simulink model "Resp"  (R2024b)
settings: Solver=ode15s  StartTime=0  StopTime=30  MaxStep=1e-3  RelTol=1e-3
libraries: slpidlib x1
settings Model: Creator=piqui
settings DataIOCC: ReturnWorkspaceOutputs=off  TimeSaveName=t
settings DebuggingCC: AlgebraicLoopMsg=none  ArtificialAlgebraicLoopMsg=none  MaxConsecutiveZCsMsg=none  OperatingPointInterfaceChecksumMismatchMsg=none
settings RTWCC: GPUComputeCapability=3.5

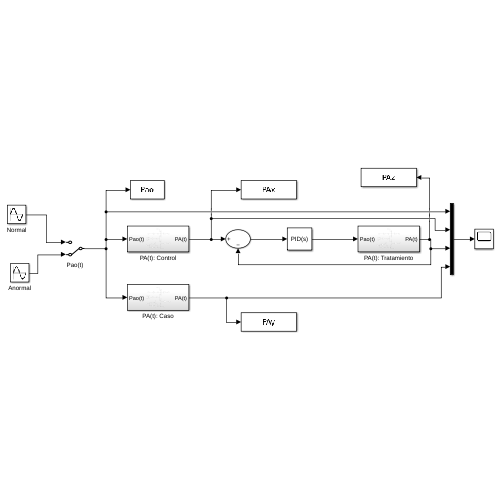
[thumbnail: Simulink's stored preview of the top-level diagram]
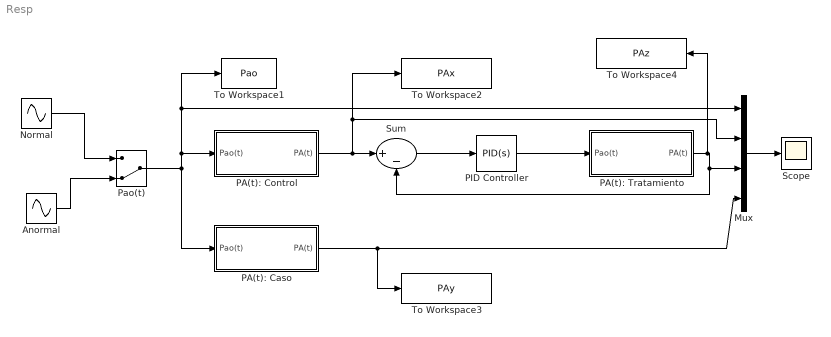
== system Resp ==
  Anormal : Sin  Amplitude=1.5  Frequency=pi/2  SampleTime=0
  Mux : Mux
  Normal : Sin  Amplitude=2.5  Frequency=pi  SampleTime=0
  PA(t): Caso : Subsystem
  PA(t): Control : Subsystem
  PA(t): Tratamiento : Subsystem
  PID Controller : slpidlib/PID Controller  Controller=PID  Form=Parallel  TimeDomain=Continuous-time  UseExternalTs=off  SampleTime=-1  IntegratorMethod=Forward Euler  FilterMethod=Forward Euler  ControllerParametersSource=internal  P=1511.4945  I=74979.6737  UseKiTs=off  D=7.0888  UseExternalDerivativeSource=off  N=55877.0023696936  UseFilter=on  TunerSelectOption=Transfer Function Based (PID Tuner App)  InitialConditionSource=internal  InitialConditionForIntegrator=0  InitialConditionForFilter=0  DifferentiatorICPrevScaledInput=0  ExternalReset=none  TrackingMode=off  Kt=1  LimitOutput=off  SatLimitsSource=internal  UpperSaturationLimit=inf  LowerSaturationLimit=-inf  LinearizeAsGain=on  AntiWindupMode=none  Kb=1  LimitIntegrator=off  UpperIntegratorSaturationLimit=inf  LowerIntegratorSaturationLimit=-inf  POutMin=[]  POutMax=[]  IOutMin=[]  IOutMax=[]  DOutMin=[]  DOutMax=[]  NOutMin=[]  NOutMax=[]  SumOutMin=[]  SumOutMax=[]  SaturationOutMin=[]  SaturationOutMax=[]  PParamMin=[]  PParamMax=[]  IParamMin=[]  IParamMax=[]  DParamMin=[]  DParamMax=[]  NParamMin=[]  NParamMax=[]  KbParamMin=[]  KbParamMax=[]  KtParamMin=[]  KtParamMax=[]  KbOutMin=[]  KbOutMax=[]  KtOutMin=[]  KtOutMax=[]  IntegratorOutMin=[]  IntegratorOutMax=[]  FilterOutMin=[]  FilterOutMax=[]  SumI1OutMin=[]  SumI1OutMax=[]  SumI2OutMin=[]  SumI2OutMax=[]  SumI3OutMin=[]  SumI3OutMax=[]  SumI4OutMin=[]  SumI4OutMax=[]  SumDOutMin=[]  SumDOutMax=[]  DifferentiatorOutMin=[]  DifferentiatorOutMax=[]  FilterDiffOutCoefMin=[]  FilterDiffOutCoefMax=[]  ReciprocalOutMin=[]  ReciprocalOutMax=[]  SumDenOutMin=[]  SumDenOutMax=[]  SumNumOutMin=[]  SumNumOutMax=[]  DivideOutMin=[]  DivideOutMax=[]  UdiffTsProdOutMin=[]  UdiffTsProdOutMax=[]  NTsProdOutMin=[]  NTsProdOutMax=[]  UintegralTsProdOutMin=[]  UintegralTsProdOutMax=[]  UngainTsProdOutMin=[]  UngainTsProdOutMax=[]  ClampingZeroOutDataTypeStr=Inherit: Inherit via back propagation  ClampingZeroOutMin=[]  ClampingZeroOutMax=[]  FilterDenConstantOutDataTypeStr=Inherit: Inherit via back propagation  FilterDenConstantOutMin=[]  FilterDenConstantOutMax=[]  PCopyOutDataTypeStr=Inherit: Inherit via back propagation  PCopyOutMin=[]  PCopyOutMax=[]  NCopyOutDataTypeStr=Inherit: Inherit via back propagation  NCopyOutMin=[]  NCopyOutMax=[]  IntegratorContinuousStateAttributes=''  IntegratorStateMustResolveToSignalObject=off  IntegratorRTWStateStorageClass=Auto  FilterContinuousStateAttributes=''  FilterStateMustResolveToSignalObject=off  FilterRTWStateStorageClass=Auto  ParallelPVariant=InternalParameters  IdealPVariant=Disabled  IVariant=InternalParameters  DVariant=InternalParameters  IntegratorVariant=Continuous  SatVariant=Disabled  AWVariant=Passthrough  PCopyVariant=Disabled  TRVariant=Disabled  FdbkBlocksVariant=Forward  IdealPFdbkVariant=Disabled  SatFdbkVariant=Disabled  DerivativeFilterVariant=ContFilter  NVariant=InternalParameters  NCopyVariant=Disabled  FilterICVariant=InternalICsFilter  IntegratorICVariant=InternalICs  ExternalResetVariant=Disabled  TRSumVariant=Passthrough  SumFdbkVariant=Disabled  SumVariant=Sum_PID  TsampFilterVariant=InternalTs  TsampNgainVariant=Passthrough  TsampIntegralVariant=Disabled_SignalSpec  ExternalSaturationOutDataTypeStr=Inherit: Same as second input  DerivativeSourceVariant=ErrorSignal  PreIntVariant=InternalPreInt
  Pao(t) : ManualSwitch  CurrentSetting=0
  Scope : Scope
  Sum : Sum  Inputs=|+-
  To Workspace1 : ToWorkspace  VariableName=Pao  SampleTime=-1
  To Workspace2 : ToWorkspace  VariableName=PAx  SampleTime=-1
  To Workspace3 : ToWorkspace  VariableName=PAy  SampleTime=-1
  To Workspace4 : ToWorkspace  VariableName=PAz  SampleTime=-1
  wires:
  Normal/1 -> Pao(t)/1
  Anormal/1 -> Pao(t)/2
  Pao(t)/1 -> PA(t): Control/1(Pao(t)), To Workspace1/1, Mux/1, PA(t): Caso/1(Pao(t))
  PA(t): Control/1(PA(t)) -> Mux/2, To Workspace2/1, Sum/1
  Sum/1 -> PID Controller/1
  PID Controller/1 -> PA(t): Tratamiento/1(Pao(t))
  PA(t): Caso/1(PA(t)) -> To Workspace3/1, Mux/4
  PA(t): Tratamiento/1(PA(t)) -> To Workspace4/1, Sum/2, Mux/3
  Mux/1 -> Scope/1

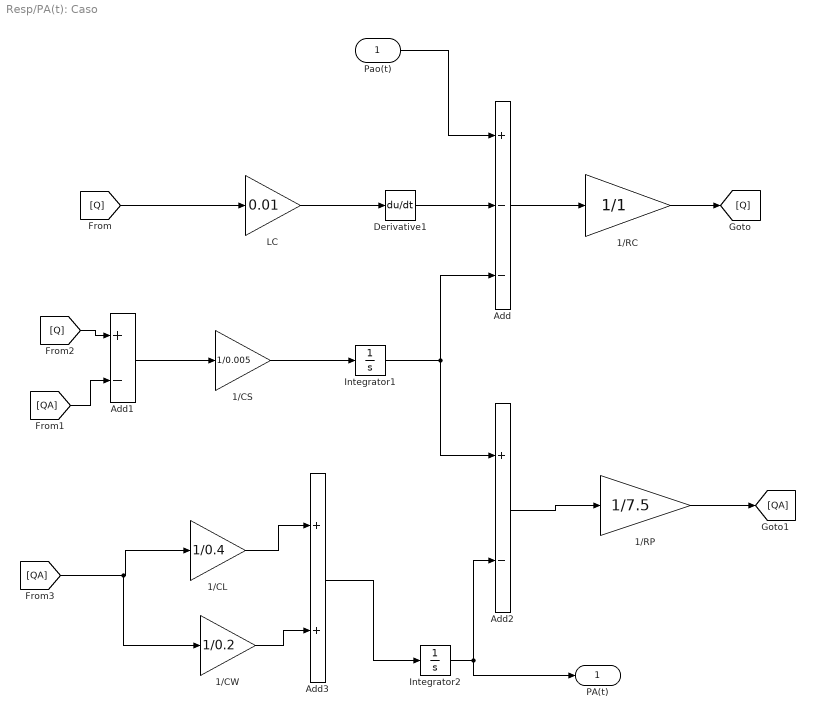
== system Resp/PA(t): Caso ==
  Pao(t) : Inport
  1/CL : Gain  Gain=1/0.4
  1/CS : Gain  Gain=1/0.005
  1/CW : Gain  Gain=1/0.2
  1/RC : Gain  Gain=1/1
  1/RP : Gain  Gain=1/7.5
  Add : Sum  Inputs=+--
  Add1 : Sum  Inputs=+-
  Add2 : Sum  Inputs=+-
  Add3 : Sum
  Derivative1 : Derivative
  Integrator1 : Integrator
  Integrator2 : Integrator
  LC : Gain  Gain=0.01
  PA(t) : Outport
  wires:
  [Q] -> Add1/1
  1/RC/1 -> [Q]
  [QA] -> Add1/2
  Add2/1 -> 1/RP/1
  [Q] -> LC/1
  Add/1 -> 1/RC/1
  1/RP/1 -> [QA]
  Pao(t)/1 -> Add/1
  LC/1 -> Derivative1/1
  Derivative1/1 -> Add/2
  Add1/1 -> 1/CS/1
  1/CS/1 -> Integrator1/1
  Integrator1/1 -> Add/3, Add2/1
  [QA] -> 1/CW/1, 1/CL/1
  1/CL/1 -> Add3/1
  1/CW/1 -> Add3/2
  Add3/1 -> Integrator2/1
  Integrator2/1 -> Add2/2, PA(t)/1

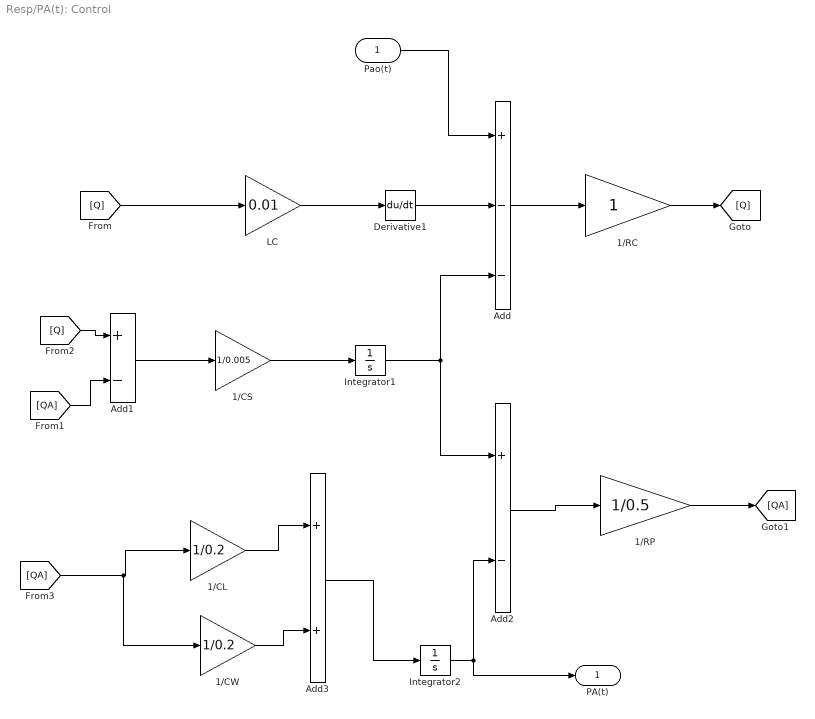
== system Resp/PA(t): Control ==
  Pao(t) : Inport
  1/CL : Gain  Gain=1/0.2
  1/CS : Gain  Gain=1/0.005
  1/CW : Gain  Gain=1/0.2
  1/RC : Gain
  1/RP : Gain  Gain=1/0.5
  Add : Sum  Inputs=+--
  Add1 : Sum  Inputs=+-
  Add2 : Sum  Inputs=+-
  Add3 : Sum
  Derivative1 : Derivative
  Integrator1 : Integrator
  Integrator2 : Integrator
  LC : Gain  Gain=0.01
  PA(t) : Outport
  wires:
  [Q] -> Add1/1
  1/RC/1 -> [Q]
  [QA] -> Add1/2
  Add2/1 -> 1/RP/1
  [Q] -> LC/1
  Add/1 -> 1/RC/1
  1/RP/1 -> [QA]
  Pao(t)/1 -> Add/1
  LC/1 -> Derivative1/1
  Derivative1/1 -> Add/2
  Add1/1 -> 1/CS/1
  1/CS/1 -> Integrator1/1
  Integrator1/1 -> Add/3, Add2/1
  [QA] -> 1/CW/1, 1/CL/1
  1/CL/1 -> Add3/1
  1/CW/1 -> Add3/2
  Add3/1 -> Integrator2/1
  Integrator2/1 -> Add2/2, PA(t)/1

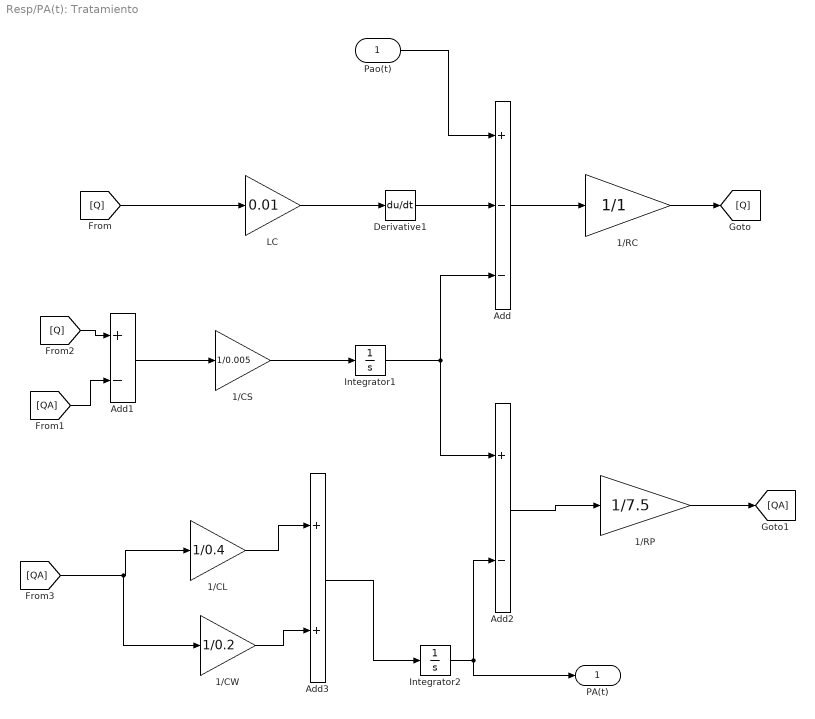
== system Resp/PA(t): Tratamiento ==
  Pao(t) : Inport
  1/CL : Gain  Gain=1/0.4
  1/CS : Gain  Gain=1/0.005
  1/CW : Gain  Gain=1/0.2
  1/RC : Gain  Gain=1/1
  1/RP : Gain  Gain=1/7.5
  Add : Sum  Inputs=+--
  Add1 : Sum  Inputs=+-
  Add2 : Sum  Inputs=+-
  Add3 : Sum
  Derivative1 : Derivative
  Integrator1 : Integrator
  Integrator2 : Integrator
  LC : Gain  Gain=0.01
  PA(t) : Outport
  wires:
  [Q] -> Add1/1
  1/RC/1 -> [Q]
  [QA] -> Add1/2
  Add2/1 -> 1/RP/1
  [Q] -> LC/1
  Add/1 -> 1/RC/1
  1/RP/1 -> [QA]
  Pao(t)/1 -> Add/1
  LC/1 -> Derivative1/1
  Derivative1/1 -> Add/2
  Add1/1 -> 1/CS/1
  1/CS/1 -> Integrator1/1
  Integrator1/1 -> Add/3, Add2/1
  [QA] -> 1/CW/1, 1/CL/1
  1/CL/1 -> Add3/1
  1/CW/1 -> Add3/2
  Add3/1 -> Integrator2/1
  Integrator2/1 -> Add2/2, PA(t)/1
